simulink model "hummel_and_hubbard"  (R2021b)
settings: Solver=VariableStepAuto  StartTime=0.0  StopTime=10.0  RelTol=1e-3
values from neighbouring files (symbols this model uses):
  amb = evalin( 'base', 'amb')    [flatball_6dof_eqom.m]
  C = evalin( 'base', 'C')    [flatball_6dof_eqom.m]
  disc = evalin( 'base', 'disc')    [flatball_6dof_eqom.m]    (also in flatball_6dof_init.m = struct; flatball_init_disc_params.m = struct)
  Y0 = [0 0 -1, 0 15*C.DEG2RAD 0, 15 0 0, 0 0 (2*15*0.29/disc.d)]    [flatball_6dof_eqom.m]
libraries: simulink x4, aerolibanim x2, aerolibnav x2, matrix_library x2, mspfiltlib x1
(part 2 of 3)

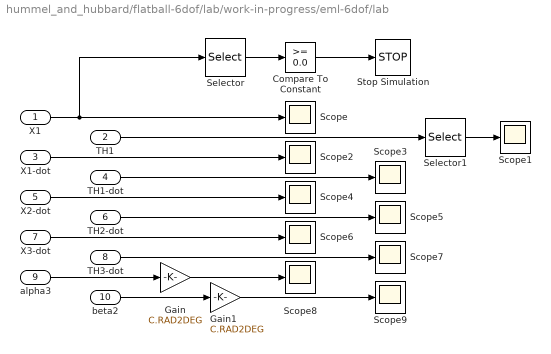
== system hummel_and_hubbard/flatball-6dof/lab/work-in-progress/eml-6dof/lab ==
  X1 : Inport
  TH1 : Inport  Port=2
  X1-dot : Inport  Port=3
  TH1-dot : Inport  Port=4
  X2-dot : Inport  Port=5
  TH2-dot : Inport  Port=6
  X3-dot : Inport  Port=7
  TH3-dot : Inport  Port=8
  alpha3 : Inport  Port=9
  beta2 : Inport  Port=10
  Compare To Constant : simulink/Logic and Bit Operations/Compare To Constant  relop=>=  const=0.0  OutDataTypeStr=boolean
  Gain : Gain  Gain=C.RAD2DEG
  Gain1 : Gain  Gain=C.RAD2DEG
  Scope{,1..9} (10 alike) : Scope
  Selector : Selector  InputPortWidth=3  IndexOptions=Index vector (dialog)  Indices=[3]  OutputSizes=1
  Selector1 : Selector  InputPortWidth=3  IndexOptions=Index vector (dialog)  Indices=[1 2]  OutputSizes=1
  Stop Simulation : Stop
  wires:
  alpha3/1 -> Gain/1
  X1-dot/1 -> Scope2/1
  X3-dot/1 -> Scope6/1
  beta2/1 -> Gain1/1
  X1/1 -> Selector/1, Scope/1
  TH1/1 -> Selector1/1
  X2-dot/1 -> Scope4/1
  TH2-dot/1 -> Scope5/1
  TH1-dot/1 -> Scope3/1
  TH3-dot/1 -> Scope7/1
  Compare To Constant/1 -> Stop Simulation/1
  Selector/1 -> Compare To Constant/1
  Gain/1 -> Scope8/1
  Gain1/1 -> Scope9/1
  Selector1/1 -> Scope1/1

== system hummel_and_hubbard/flatball-6dof/calc-F-M/lab/calc-F/aero-coeff/Subsystem ==
  alpha : Inport
  Cd0 : Constant  Value=disc.CD0
  Cda : Constant  Value=disc.CDa
  Product : Product
  Square : Math  Operator=square  SaturateOnIntegerOverflow=on
  Sum : Sum
  Sum1 : Sum
  alpha0 : Constant  Value=disc.alpha0
  Cd : Outport
  wires:
  Sum1/1 -> Cd/1
  Square/1 -> Product/2
  Product/1 -> Sum1/2
  Cda/1 -> Product/1
  Cd0/1 -> Sum1/1
  Sum/1 -> Square/1
  alpha0/1 -> Sum/2
  alpha/1 -> Sum/1

== system hummel_and_hubbard/flatball-6dof/calc-F-M/lab/calc-F/aero-coeff/Subsystem1 ==
  alpha : Inport
  CL0 : Constant  Value=disc.CL0
  CLa : Constant  Value=disc.CLa
  Product : Product
  Sum1 : Sum
  Cl : Outport
  wires:
  alpha/1 -> Product/2
  CL0/1 -> Sum1/1
  CLa/1 -> Product/1
  Product/1 -> Sum1/2
  Sum1/1 -> Cl/1

== system hummel_and_hubbard/flatball-6dof/calc-F-M/lab/calc-M/aero-coeff/Subsystem2 ==
  alpha : Inport
  CM0 : Constant  Value=disc.CM0
  CMa : Constant  Value=disc.CMa
  Product : Product
  Sum1 : Sum
  Cm : Outport
  wires:
  Sum1/1 -> Cm/1
  Product/1 -> Sum1/2
  CMa/1 -> Product/1
  CM0/1 -> Sum1/1
  alpha/1 -> Product/2

== system hummel_and_hubbard/flatball-6dof/calc-F-M/lab/helpers/Subsystem1/transformation-matrices ==
  TH : Inport
  Ta : MATLAB Function  TreatAsAtomicUnit=on
  Tr : MATLAB Function  TreatAsAtomicUnit=on
  Ta12 : Outport
  Tr12 : Outport  Port=2
  wires:
  TH/1 -> Ta/1(TH), Tr/1(TH)
  Ta/1(M) -> Ta12/1  "Ta12"
  Tr/1(M) -> Tr12/1  "Tr12"

== system hummel_and_hubbard/flatball-6dof/calc-F-M/lab/wrk/c&p/Subsystem1 ==
  X1_dot : Inport
  TH1 : Inport  Port=2
  TH1_dot : Inport  Port=3
  MatrixMultiply : Product  Multiplication=Matrix(*)
  MatrixMultiply1 : Product  Multiplication=Matrix(*)
  Transpose : Math  Operator=transpose  SaturateOnIntegerOverflow=on
  Transpose1 : Math  Operator=transpose  SaturateOnIntegerOverflow=on
  transformation-matrices : Subsystem
  w_ : MATLAB Function  TreatAsAtomicUnit=on
  TH2_dot : Outport
  w~ : Outport  Port=2
  X2_dot : Outport  Port=3
  Ta12 : Outport  Port=4
  wires:
  MatrixMultiply/1 -> X2_dot/1
  MatrixMultiply1/1 -> w_/1(THdot), TH2_dot/1
  transformation-matrices/1(Ta12) -> Transpose/1, Ta12/1
  transformation-matrices/2(Tr12) -> Transpose1/1
  X1_dot/1 -> MatrixMultiply/2
  TH1_dot/1 -> MatrixMultiply1/2
  TH1/1 -> transformation-matrices/1(TH)
  w_/1(M) -> w~/1  "w_"
  Transpose/1 -> MatrixMultiply/1  "Ta21"
  Transpose1/1 -> MatrixMultiply1/1  "Ta21"

== system hummel_and_hubbard/flatball-6dof/calc-F-M/lab/wrk/c&p/aero-coeff ==
  alpha : Inport
  Subsystem : Subsystem
  Subsystem1 : Subsystem
  Subsystem2 : Subsystem
  Cd : Outport
  Cl : Outport  Port=2
  Cm : Outport  Port=3
  wires:
  alpha/1 -> Subsystem2/1(alpha), Subsystem1/1(alpha), Subsystem/1(alpha)
  Subsystem2/1(Cm) -> Cm/1
  Subsystem1/1(Cl) -> Cl/1
  Subsystem/1(Cd) -> Cd/1

== system hummel_and_hubbard/flatball-6dof/calc-F-M/lab/wrk/c&p/q-inf ==
  x1dt : Inport
  Gain : Gain  Gain=0.5
  Product1 : Product  Inputs=3
  S : Constant  Value=disc.A
  Square : Math  Operator=square  SaturateOnIntegerOverflow=on
  rho : Constant  Value=amb.rho
  vector-norm : MATLAB Function  TreatAsAtomicUnit=on
  q-inf-S : Outport
  wires:
  Product1/1 -> Gain/1
  rho/1 -> Product1/3
  x1dt/1 -> vector-norm/1(vec)
  vector-norm/1(norm) -> Square/1
  S/1 -> Product1/2
  Square/1 -> Product1/1
  Gain/1 -> q-inf-S/1

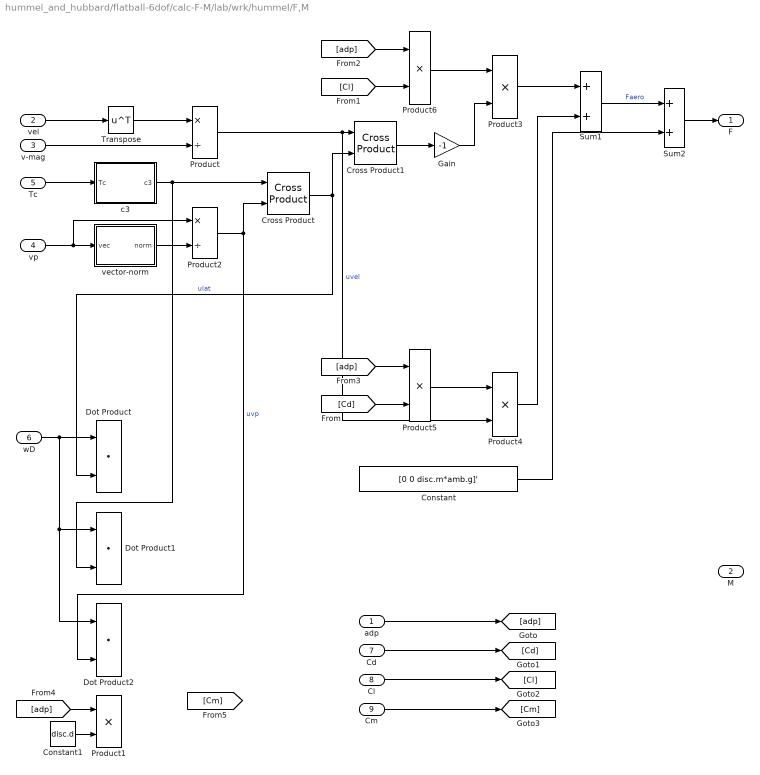
== system hummel_and_hubbard/flatball-6dof/calc-F-M/lab/wrk/hummel/F,M ==
  adp : Inport
  vel : Inport  Port=2
  v-mag : Inport  Port=3
  vp : Inport  Port=4
  Tc : Inport  Port=5
  wD : Inport  Port=6
  Cd : Inport  Port=7
  Cl : Inport  Port=8
  Cm : Inport  Port=9
  Constant : Constant  Value=[0 0 disc.m*amb.g]'
  Constant1 : Constant  Value=disc.d
  Cross Product : matrix_library/Cross Product
      settings: SourceProductBaseCode=SL
  Cross Product1 : matrix_library/Cross Product
      settings: SourceProductBaseCode=SL
  Dot Product : DotProduct  InputSameDT=on  OutDataTypeStr=Inherit: Inherit via internal rule
  Dot Product1 : DotProduct  InputSameDT=on  OutDataTypeStr=Inherit: Inherit via internal rule
  Dot Product2 : DotProduct  InputSameDT=on  OutDataTypeStr=Inherit: Inherit via internal rule
  Gain : Gain  Gain=-1
  Product : Product  Inputs=*/
  Product1 : Product  Inputs=**
  Product2 : Product  Inputs=*/
  Product{3..6} (4 alike) : Product
  Sum1 : Sum
  Sum2 : Sum
  Transpose : Math  Operator=transpose  SaturateOnIntegerOverflow=on
  c3 : MATLAB Function  TreatAsAtomicUnit=on
  vector-norm : MATLAB Function  TreatAsAtomicUnit=on
  F : Outport
  M : Outport  Port=2
  wires:
  vel/1 -> Transpose/1
  v-mag/1 -> Product/2
  vp/1 -> Product2/1, vector-norm/1(vec)
  vector-norm/1(norm) -> Product2/2
  Product2/1 -> Dot Product2/2, Cross Product/2  "uvp"
  Tc/1 -> c3/1(Tc)
  c3/1(c3) -> Dot Product1/2, Cross Product/1
  Cross Product/1 -> Cross Product1/2, Dot Product/2  "ulat"
  Product/1 -> Cross Product1/1, Product4/2  "uvel"
  Cross Product1/1 -> Gain/1
  Gain/1 -> Product3/2
  Product3/1 -> Sum1/1
  Product4/1 -> Sum1/2
  Sum1/1 -> Sum2/1  "Faero"
  Transpose/1 -> Product/1
  Sum2/1 -> F/1
  Constant/1 -> Sum2/2
  adp/1 -> [adp]
  Constant1/1 -> Product1/2
  wD/1 -> Dot Product2/1, Dot Product1/1, Dot Product/1
  Product5/1 -> Product4/1
  [Cl] -> Product6/2
  [Cd] -> Product5/2
  Product6/1 -> Product3/1
  [adp] -> Product6/1
  [adp] -> Product5/1
  Cd/1 -> [Cd]
  Cl/1 -> [Cl]
  Cm/1 -> [Cm]
  [adp] -> Product1/1

== system hummel_and_hubbard/flatball-6dof/calc-F-M/lab/wrk/hummel/Radv ==
  v-mag : Inport
  TH-dt : Inport  Port=2
  Gain : Gain  Gain=0.5
  Product1 : Product  Inputs=**/
  Selector : Selector  InputPortWidth=3  IndexOptions=Index vector (dialog)  Indices=[3]  OutputSizes=1
  "[0.5 .. inf]" : Saturate  UpperLimit=inf  LowerLimit=0.50
  d : Constant  Value=disc.d
  Radv : Outport
  wires:
  Product1/1 -> Radv/1
  d/1 -> Gain/1
  TH-dt/1 -> Selector/1
  Selector/1 -> Product1/1
  Gain/1 -> Product1/2
  v-mag/1 -> "[0.5 .. inf]"/1
  "[0.5 .. inf]"/1 -> Product1/3

== system hummel_and_hubbard/flatball-6dof/calc-F-M/lab/wrk/hummel/Subsystem ==
  phi : Inport
  theta : Inport  Port=2
  Tc : MATLAB Function  TreatAsAtomicUnit=on
  T : Outport
  wires:
  theta/1 -> Tc/2(theta)
  phi/1 -> Tc/1(phi)
  Tc/1(Tc) -> T/1

== system hummel_and_hubbard/flatball-6dof/calc-F-M/lab/wrk/hummel/adp ==
  v-mag : Inport
  A : Constant  Value=disc.A
  Gain : Gain  Gain=0.5
  Product : Product
  Product1 : Product  Inputs=3
  rho : Constant  Value=amb.rho
  adp : Outport
  wires:
  Product1/1 -> adp/1
  rho/1 -> Product/1
  A/1 -> Product/2
  Product/1 -> Gain/1
  v-mag/1 -> Product1/2, Product1/1
  Gain/1 -> Product1/3

== system hummel_and_hubbard/flatball-6dof/calc-F-M/lab/wrk/hummel/aero-coeff ==
  alpha : Inport
  Subsystem : Subsystem
  Subsystem1 : Subsystem
  Subsystem2 : Subsystem
  Cd : Outport
  Cl : Outport  Port=2
  Cm : Outport  Port=3
  wires:
  alpha/1 -> Subsystem2/1(alpha), Subsystem1/1(alpha), Subsystem/1(alpha)
  Subsystem2/1(Cm) -> Cm/1
  Subsystem1/1(Cl) -> Cl/1
  Subsystem/1(Cd) -> Cd/1

== system hummel_and_hubbard/flatball-6dof/calc-F-M/lab/wrk/c&p/Subsystem1/transformation-matrices ==
  TH : Inport
  Ta : MATLAB Function  TreatAsAtomicUnit=on
  Tr : MATLAB Function  TreatAsAtomicUnit=on
  Ta12 : Outport
  Tr12 : Outport  Port=2
  wires:
  TH/1 -> Ta/1(TH), Tr/1(TH)
  Ta/1(Ta12) -> Ta12/1
  Tr/1(Tr12) -> Tr12/1

== system hummel_and_hubbard/flatball-6dof/calc-F-M/lab/wrk/c&p/aero-coeff/Subsystem ==
  alpha : Inport
  Cd0 : Constant  Value=disc.CD0
  Cda : Constant  Value=disc.CDa
  Product : Product
  Square : Math  Operator=square  SaturateOnIntegerOverflow=on
  Sum : Sum
  Sum1 : Sum
  alpha0 : Constant  Value=disc.alpha0
  Cd : Outport
  wires:
  Sum1/1 -> Cd/1
  Square/1 -> Product/2
  Product/1 -> Sum1/2
  Cda/1 -> Product/1
  Cd0/1 -> Sum1/1
  Sum/1 -> Square/1
  alpha0/1 -> Sum/2
  alpha/1 -> Sum/1

== system hummel_and_hubbard/flatball-6dof/calc-F-M/lab/wrk/c&p/aero-coeff/Subsystem1 ==
  alpha : Inport
  CL0 : Constant  Value=disc.CL0
  CLa : Constant  Value=disc.CLa
  Product : Product
  Sum1 : Sum
  Cl : Outport
  wires:
  alpha/1 -> Product/2
  CL0/1 -> Sum1/1
  CLa/1 -> Product/1
  Product/1 -> Sum1/2
  Sum1/1 -> Cl/1

== system hummel_and_hubbard/flatball-6dof/calc-F-M/lab/wrk/c&p/aero-coeff/Subsystem2 ==
  alpha : Inport
  CM0 : Constant  Value=disc.CM0
  CMa : Constant  Value=disc.CMa
  Product : Product
  Sum1 : Sum
  Cm : Outport
  wires:
  Sum1/1 -> Cm/1
  Product/1 -> Sum1/2
  CMa/1 -> Product/1
  CM0/1 -> Sum1/1
  alpha/1 -> Product/2

== system hummel_and_hubbard/flatball-6dof/calc-F-M/lab/wrk/hummel/aero-coeff/Subsystem ==
  alpha : Inport
  Cd0 : Constant  Value=disc.CD0
  Cda : Constant  Value=disc.CDa
  Product : Product
  Square : Math  Operator=square  SaturateOnIntegerOverflow=on
  Sum : Sum
  Sum1 : Sum
  alpha0 : Constant  Value=disc.alpha0
  Cd : Outport
  wires:
  Sum1/1 -> Cd/1
  Square/1 -> Product/2
  Product/1 -> Sum1/2
  Cda/1 -> Product/1
  Cd0/1 -> Sum1/1
  Sum/1 -> Square/1
  alpha0/1 -> Sum/2
  alpha/1 -> Sum/1

== system hummel_and_hubbard/flatball-6dof/calc-F-M/lab/wrk/hummel/aero-coeff/Subsystem1 ==
  alpha : Inport
  CL0 : Constant  Value=disc.CL0
  CLa : Constant  Value=disc.CLa
  Product : Product
  Sum1 : Sum
  Cl : Outport
  wires:
  alpha/1 -> Product/2
  CL0/1 -> Sum1/1
  CLa/1 -> Product/1
  Product/1 -> Sum1/2
  Sum1/1 -> Cl/1

== system hummel_and_hubbard/flatball-6dof/calc-F-M/lab/wrk/hummel/aero-coeff/Subsystem2 ==
  alpha : Inport
  CM0 : Constant  Value=disc.CM0
  CMa : Constant  Value=disc.CMa
  Product : Product
  Sum1 : Sum
  Cm : Outport
  wires:
  Sum1/1 -> Cm/1
  Product/1 -> Sum1/2
  CMa/1 -> Product/1
  CM0/1 -> Sum1/1
  alpha/1 -> Product/2

== matlab function hummel_and_hubbard/flatball-6dof/calc-F-M/lab/helpers/Subsystem2/angle-of-attack ==
  data: Xdot input; alpha output
function alpha  = f( Xdot)
% calculate angle of attack

alpha = atan( Xdot(3) / Xdot(1));

== matlab function hummel_and_hubbard/flatball-6dof/calc-Xdot/calc-Xdot ==
  data: X input; F input; Xdot output
function Xdot   = f_lin( X, F)
% flatball equations of motion - NED (north-east-down) configuration
%

%% internal states
% x = X(1); y = X(2); z = X(3);
u = X(7); v = X(8); w = X(9);

Xdot = zeros(1,6);

%% define non-aerodynamic parameters
disc = struct;
disc.m = 0.175; % Kg

%%
    xdotdot = F(1) / disc.m;
    ydotdot = F(2) / disc.m;
    zdotdot = F(3) / disc.m;

%%
Xdot(1) = u;
Xdot(2) = v;
Xdot(3) = w;

Xdot(4) = xdotdot;
Xdot(5) = ydotdot;
Xdot(6) = zdotdot;

== matlab function hummel_and_hubbard/flatball-6dof/calc-F-M/lab/wrk/hummel/vector-norm ==
  data: vec input; norm output
function norm = fcn( vec)

norm = sqrt( vec(1)*vec(1) + vec(2)*vec(2) + vec(3)*vec(3));

== matlab function hummel_and_hubbard/flatball-6dof/calc-F-M/lab/wrk/hummel/Subsystem/Tc ==
  data: phi input; theta input; Tc output
function Tc = fcn( phi, theta)

sin_theta = sin( theta);
cos_theta = cos( theta);
sin_phi = sin( phi);
cos_phi = cos(phi);

Tc = [
    cos_theta sin_theta*sin_phi -sin_theta*cos_phi;
    0 cos_phi sin_phi;
    sin_theta -cos_theta*sin_phi cos_theta*cos_phi;
    ];

== matlab function hummel_and_hubbard/flatball-6dof/calc-F-M/lab/wrk/hummel/vp ==
  data: vel input; vp output; Tc input; vc3 input
function vp = fcn( vel, Tc, vc3)

c3 = Tc(:,3);

vp = [ vel - vc3*c3];

== matlab function hummel_and_hubbard/flatball-6dof/calc-F-M/lab/wrk/hummel/alpha ==
  data: v_N input; vc3 input; alpha output
function alpha = fcn( v_N, vc3)

alpha = atan( vc3 / norm( v_N)); % angle of attack

== matlab function hummel_and_hubbard/flatball-6dof/calc-F-M/lab/wrk/hummel/vc3 ==
  data: vel input; vc3 output; Tc input
function vc3 = fcn( vel, Tc)

c3 = Tc(:,3);
vc3 = dot( vel, c3);

== matlab function hummel_and_hubbard/flatball-6dof/calc-F-M/lab/wrk/c&p/Ta ==
  data: beta input; T output
function T  = Ta23( beta)
% transformation matrix
%

cos_beta = cos( beta);
sin_beta = sin( beta);

T = [ ...
    cos_beta -sin_beta 0;
    -sin_beta cos_beta 0;
    0 0 1;
    ];

== matlab function hummel_and_hubbard/flatball-6dof/calc-F-M/lab/wrk/hummel/F,M/vector-norm ==
  data: vec input; norm output
function norm = fcn( vec)

norm = sqrt( vec(1)*vec(1) + vec(2)*vec(2) + vec(3)*vec(3));

== matlab function hummel_and_hubbard/flatball-6dof/calc-F-M/lab/wrk/hummel/F,M/c3 ==
  data: Tc input; c3 output
function c3 = fcn( Tc)

c3 = Tc(:,3);

== matlab function hummel_and_hubbard/flatball-6dof/calc-F-M/lab/wrk/hummel/wD ==
  data: TH input; TH_dt input; wD output; Tc input
function wD = fcn( TH, TH_dt, Tc)

cos_theta = cos( TH(2));
sin_theta = sin( TH(2));

phidot = TH_dt(1);
thetadot = TH_dt(2);
gammadot = TH_dt(3);

wD_N_inC = [phidot*cos_theta thetadot phidot*sin_theta+gammadot];
wD = Tc' * wD_N_inC';

== matlab function hummel_and_hubbard/flatball-6dof/calc-F-M/lab/wrk/c&p/q-inf/vector-norm ==
  data: vec input; norm output
function norm = fcn( vec)

norm = sqrt( vec(1)*vec(1) + vec(2)*vec(2) + vec(3)*vec(3));

== matlab function hummel_and_hubbard/flatball-6dof/calc-F-M/lab/wrk/c&p/Subsystem1/transformation-matrices/Ta ==
  data: TH input; Ta12 output
function Ta12  = Ta( TH)
% transformation matrix
%
phi = TH(1); theta = TH(2); psi = TH(3);

cos_phi = cos( phi);
cos_theta = cos( theta);
cos_psi = cos( psi);

sin_phi = sin( phi);
sin_theta = sin( theta);
sin_psi = sin( psi);

Ta12 = [ ...
    cos_theta*cos_psi sin_phi*sin_theta*cos_phi-cos_phi*sin_psi cos_phi*sin_theta*cos_psi+sin_phi*sin_psi;
    cos_theta*sin_psi sin_phi*sin_theta*sin_psi+cos_phi*cos_psi cos_phi*sin_theta*sin_psi-sin_phi*cos_psi;
    -sin_theta sin_phi*cos_theta cos_phi*cos_theta
    ];

% cos_neg_phi = cos( -phi);
% cos_neg_theta = cos( -theta);
% cos_neg_psi = cos( -psi);
% 
% sin_neg_phi = sin( -phi);
% sin_neg_theta = sin( -theta);
% sin_neg_psi = sin( -psi);
% 
% Ta12 = [ ...
%     cos_neg_theta*cos_neg_psi sin_neg_phi*sin_neg_theta*cos_neg_phi-cos_neg_phi*sin_neg_psi cos_neg_phi*sin_neg_theta*cos_neg_psi+sin_neg_phi*sin_neg_psi;
%     cos_neg_theta*sin_neg_psi sin_neg_phi*sin_neg_theta*sin_neg_psi+cos_neg_phi*cos_neg_psi cos_neg_phi*sin_neg_theta*sin_neg_psi-sin_neg_phi*cos_neg_psi;
%     -sin_neg_theta sin_neg_phi*cos_neg_theta cos_neg_phi*cos_neg_theta
%     ];

== matlab function hummel_and_hubbard/flatball-6dof/calc-F-M/lab/wrk/c&p/Subsystem1/transformation-matrices/Tr ==
  data: TH input; Tr12 output
function Tr12  = Tr( TH)
% transformation matrix
%
phi = TH(1); theta = TH(2); psi = TH(3);

cos_phi = cos( phi);
cos_theta = cos( theta);
cos_psi = cos( psi);

sin_phi = sin( phi);
sin_theta = sin( theta);
sin_psi = sin( psi);

Tr12 = [
    1 0 -sin_theta;
    0 cos_phi cos_theta*sin_psi;
    0 -sin_phi cos_theta*cos_psi;
    ];

== matlab function hummel_and_hubbard/flatball-6dof/calc-F-M/lab/wrk/c&p/Subsystem1/w_ ==
  data: THdot input; M output
function M  = w_( THdot)
% transformation matrix
%
p = THdot(1); q = THdot(2); r = THdot(3);

M = [ ...
    0 -r q;
    r 0 -p;
    -q p 0
    ];

== matlab function hummel_and_hubbard/flatball-6dof/calc-F-M/lab/wrk/c&p/Ta1 ==
  data: alpha input; T output
function T  = Ta34( alpha)
% transformation matrix
%

cos_alpha = cos( alpha);
sin_alpha = sin( alpha);

T= [ ...
    cos_alpha 0 -sin_alpha;
    0 1 0;
    sin_alpha 0 cos_alpha;
    ];

== matlab function hummel_and_hubbard/flatball-6dof/calc-F-M/lab/wrk/c&p/angle-of-attack ==
  data: Xdot input; alpha output
function alpha  = f( Xdot)
% calculate angle of attack

alpha = atan2( Xdot(3) / Xdot(1));

== matlab function hummel_and_hubbard/flatball-6dof/calc-F-M/lab/wrk/c&p/zero-side-slip-angle ==
  data: Xdot input; beta output
function beta  = f( Xdot)
% calculate side-slip angle

y = Xdot(2);
x = Xdot(1);

beta = atan2( y / x);

== matlab function hummel_and_hubbard/flatball-6dof/calc-F-M/lab/wrk/flatball_6dof_v1p1 ==
  data: X input; Xdot output; lift output; drag output; alpha output; AdvR output; E_trans output; E_rot output
function [Xdot, lift, drag, alpha, AdvR, E_trans, E_rot]  = flatball_6dof_eom( X)
% flatball equations of motion - NED (north-east-down) configuration
%

%% internal states
x = X(1); y = X(2); z = X(3);
xdot = X(4); ydot = X(5); zdot = X(6);

phi = X(7); theta = X(8); gamma = X(9);
phidot = X(10); thetadot = X(11); gammadot = X(12);

Xdot = zeros(1,12);

%% define ambient parameters
amb.g = 9.81; % m/s^2
amb.rho = 1.23; % Kg/m^3

%% define non-aerodynamic parameters
disc = struct;
disc.m = 0.175; % Kg
disc.A = 0.057; % m^2
disc.d = 2*sqrt(0.057/pi); % 2*sqrt(disc.A/pi); % diameter
disc.Ia = 0.002352; % moment of inertia about the spinning axis
disc.Id = 0.001219; % moment of inertia about the planar axis'

%% crowther and potts - per hummel and hubbard
% disc.CL0 = 0.13;
% disc.CLa = 3.09;
% disc.CD0 = 0.085;
% disc.CDa = 3.30;
% disc.CM0 = -0.01;
% disc.CMa = 0.057;
% 
% disc.CMq = 0.0008; % NOTE: not used
% disc.CLr = 0.0004;
% disc.CLp = -0.013;
% disc.CNr = -2.8e-5;
% 
% disc.alpha0 = -0.052; % rad

%% hummel and hubbard 2014
disc.CL0 = 0.188;
disc.CLa = 2.37;

disc.CD0 = 0.15;
disc.CDa = 1.24;

disc.CM0 = -0.06;
disc.CMa = 0.38;

disc.CMq = 0.0008; % NOTE: not used
disc.CLr = 0.0004;

disc.CNr = -2.8e-5;

disc.CLp = -0.013;

% disc.CRr = 1.4e-2; % NOTE: missing from 2014, borrowed from 2003 thesis
% disc.CRr = 3e-3; % NOTE: missing from 2014, borrowed from P&C
disc.CRr = 0.00171; % appendix of hummel thesis
disc.CRp =-5.5e-3; % NOTE: missing from 2014, borrowed from P&C

% not sure where these are from...
% disc.CMq= -1.44E-02;
% disc.CRp =-1.25E-02;
% disc.CNr = -3.41E-05; % long flight f2302

disc.alpha0 = -0.052; % rad

%% helper variables
sin_theta = sin( theta);
cos_theta = cos( theta);
sin_phi = sin( phi);
cos_phi = cos(phi);

% c = T_c_N * N --> transformation matrix T_c_N in N reference frame
T_c_N = [cos_theta sin_theta*sin_phi -sin_theta*cos_phi;
    0 cos_phi sin_phi;
    sin_theta -cos_theta*sin_phi cos_theta*cos_phi];
% c1 = T_c_N(1,:);
% c2 = T_c_N(2,:);
c3 = T_c_N(3,:);

%% aerodynamic forces and moments in N reference frame
vel = [xdot ydot zdot];
vmag = norm( vel);
vc3 = dot( vel, c3);
v_N = [ vel - vc3*c3];
Adp = 0.5 * disc.A * amb.rho * vmag*vmag;
uvel = vel / vmag;
uv_N = v_N / norm( v_N);
u_lat = cross( c3, uv_N);

wD_N_inC = [phidot*cos_theta thetadot phidot*sin_theta+gammadot];
wD_N_inN = T_c_N' * wD_N_inC';

w_v_N = dot( wD_N_inN, uv_N);
w_lat = dot( wD_N_inN, u_lat);
w_spin = dot( wD_N_inN, c3);

alpha = atan( vc3 / norm( v_N)); % angle of attack
AdvR = disc.d * w_spin / 2 / vmag; % advance ratio
E_trans = 0.5 * disc.m * vmag*vmag; % translational energy
E_rot = 0.5 * disc.Ia * gammadot*gammadot; % rotational energy

%% hacks
k_spin_down_decay = 0.25;
% k_CL_gain = 1.0; %2.5;
% k_CD_gain = 1.0; %1.5;
% k_M_gain = 1.0;

%% coefficients - f(alpha)
dalpha = alpha - disc.alpha0;
CL = disc.CL0 + disc.CLa * alpha;
CD = disc.CD0 + disc.CDa * dalpha*dalpha;
CM = disc.CM0 + disc.CMa * alpha;
Mv_N = Adp * disc.d * (sqrt(disc.d/amb.g)*disc.CRr*w_spin + disc.CRp*w_v_N) * uv_N;

%% coefficients - lookup based
% 
% CL = interp1( disc.CL_data(:,1), disc.CL_data(:,2).*k_CL_gain, alpha, 'spline');
% CD = interp1( disc.CD_data(:,1), disc.CD_data(:,2).*k_CD_gain, alpha, 'spline');
% CM = interp1( disc.CM_data(:,1), disc.CM_data(:,2).*k_M_gain, alpha, 'spline');
% % CRr = interp2( disc.CRr_rad, disc.CRr_AdvR, disc.CRr_data, alpha, AdvR,'spline');
% Mv_N = Adp * disc.d * ( disc.CRr* + disc.CRp*w_v_N) * uv_N;

%%
lift = CL * Adp;
drag = CD * Adp;
ulift = -cross( uvel, u_lat);
udrag = -uvel;
Faero = lift*ulift + drag*udrag;
Fg_N = [0 0 disc.m*amb.g]';

F = Faero' + Fg_N;

Mlat = Adp * disc.d * (CM + disc.CMq * w_lat) * u_lat;
Mspin = [0 0 disc.CNr*w_spin];
M = T_c_N * Mv_N' + T_c_N*Mlat' + Mspin';

%%
xdotdot = F(1) / disc.m;
ydotdot = F(2) / disc.m;
zdotdot = F(3) / disc.m;

phidotdot = (M(1) + disc.Id*thetadot*phidot*sin_theta - disc.Ia*thetadot*(phidot*sin_theta+gammadot) + disc.Id*thetadot*phidot*sin_theta)/disc.Id/cos_theta; 
thetadotdot = (M(2) + disc.Ia*phidot*cos_theta*(phidot*sin_theta +gammadot) - disc.Id*phidot*phidot*cos_theta*sin_theta)/disc.Id;
gammadotdot = (M(3) - disc.Ia*(k_spin_down_decay*gammadot*sin_theta + thetadot*phidot*cos_theta))/disc.Ia;

% bug in hummels report?
% gammadotdot = (M(3) - disc.Ia*(phidotdot*sin_theta + thetadot*phidot*cos_theta))/disc.Ia;
% bug in hummels report?
% w/phidotdot term, there is no decay in gammadot
% w/out gammadot term - there is no decay in gammadot
% NOTE: w/it, the decay is too agressive
% FIXME: investigate why this term is necessary for more appropriate
% spindown (based on my data)

%%
Xdot(1) = xdot;
Xdot(2) = ydot;
Xdot(3) = zdot;

Xdot(4) = xdotdot;
Xdot(5) = ydotdot;
Xdot(6) = zdotdot;

Xdot(7) = phidot;
Xdot(8) = thetadot;
Xdot(9) = gammadot;

Xdot(10) = phidotdot;
Xdot(11) = thetadotdot;
Xdot(12) = gammadotdot;

== matlab function hummel_and_hubbard/flatball-6dof/calc-F-M/lab/rotations/X-to-T_c_N ==
  data: X input; T_c_N output
function T_c_N  = f( X)
%% internal states
phi = X(7); theta = X(8);

%% helper variables
sin_theta = sin( theta);
cos_theta = cos( theta);
sin_phi = sin( phi);
cos_phi = cos(phi);

T_c_N = [
    cos_theta sin_theta*sin_phi -sin_theta*cos_phi;
    0 cos_phi sin_phi;
    sin_theta -cos_theta*sin_phi cos_theta*cos_phi
    ];

== matlab function hummel_and_hubbard/flatball-6dof/calc-F-M/lab/alpha- ==
  data: X input; alpha output; T_c_N input
function alpha  = f( X, T_c_N)
%% internal states
xdot = X(4); ydot = X(5); zdot = X(6);

%% helper variables
T_c_Npsi = T_c_N(3,:);

vel = [xdot ydot zdot];
vc3 = dot( vel, T_c_Npsi);
v_N = [ vel - vc3*T_c_Npsi];

alpha = atan( vc3 / norm( v_N)); % angle of attack

== matlab function hummel_and_hubbard/flatball-6dof/calc-F-M/lab/rotations/X-to-wD_N_inC ==
  data: X input; wD_N_inC output
function wD_N_inC  = f( X)
%% internal states
theta = X(8);
phidot = X(10); thetadot = X(11); gammadot = X(12);

%% helper variables
sin_theta = sin( theta);
cos_theta = cos( theta);

wD_N_inC = [phidot*cos_theta thetadot phidot*sin_theta+gammadot];

== matlab function hummel_and_hubbard/flatball-6dof/calc-F-M/lab/calc-F/q-inf/vector-norm ==
  data: vec input; norm output
function norm = fcn( vec)

norm = sqrt( vec(1)*vec(1) + vec(2)*vec(2) + vec(3)*vec(3));

== matlab function hummel_and_hubbard/flatball-6dof/calc-F-M/lab/calc-F/q-inf/X-to-vel ==
  data: X input; vel output
function vel = fcn( X)
xdot = X(4); ydot = X(5); zdot = X(6);
vel = [xdot ydot zdot];

== matlab function hummel_and_hubbard/flatball-6dof/calc-F-M/lab/calc-F/X-to-vel ==
  data: X input; vel output
function vel = fcn( X)
xdot = X(4); ydot = X(5); zdot = X(6);
vel = [xdot ydot zdot];

== matlab function hummel_and_hubbard/flatball-6dof/calc-F-M/lab/calc-M/X-to-vel ==
  data: X input; vel output
function vel = fcn( X)
xdot = X(4); ydot = X(5); zdot = X(6);
vel = [xdot ydot zdot];

== matlab function hummel_and_hubbard/flatball-6dof/calc-F-M/lab/calc-F/calc-F ==
  data: vel input; F output; T_c_N input; Fg_N input; CLift input; CDrag input; q_inf_times_S input
function F = fcn( vel, T_c_N, Fg_N, CLift, CDrag, q_inf_times_S)
%%
T_c_Npsi = T_c_N(3,:);

vc3 = dot( vel, T_c_Npsi);
v_N = [ vel - vc3*T_c_Npsi];
vmag = norm( vel);
uvel = vel / vmag;
uv_N = v_N / norm( v_N);
u_lat = cross( T_c_Npsi, uv_N);

lift = CLift * q_inf_times_S;
ulift = -cross( uvel, u_lat);

drag = CDrag * q_inf_times_S;
udrag = -uvel;

Faero = lift*ulift + drag*udrag;

F = Faero' + Fg_N;

== matlab function hummel_and_hubbard/flatball-6dof/calc-F-M/lab/wrk/flatball_6dof_v1p0 ==
  data: X input; Xdot output; lift output; drag output; alpha output; AdvR output; E_trans output; E_rot output
function [Xdot, lift, drag, alpha, AdvR, E_trans, E_rot]  = flatball_6dof_eom( X)
% flatball equations of motion - NED (north-east-down) configuration
%

%% internal states
x = X(1); y = X(2); z = X(3);
xdot = X(4); ydot = X(5); zdot = X(6);

phi = X(7); theta = X(8); gamma = X(9);
phidot = X(10); thetadot = X(11); gammadot = X(12);

Xdot = zeros(1,12);

%% define ambient parameters
amb.g = 9.81; % m/s^2
amb.rho = 1.23; % Kg/m^3

%% define non-aerodynamic parameters
disc = struct;
disc.m = 0.175; % Kg
disc.A = 0.057; % m^2
disc.d = 2*sqrt(0.057/pi); % 2*sqrt(disc.A/pi); % diameter
disc.Ia = 0.002352; % moment of inertia about the spinning axis
disc.Id = 0.001219; % moment of inertia about the planar axis'

disc.alpha0 = -0.052; %-4 * pi/180.0;

%% THE THREE ESTIMATED COEFFICIENTS
disc.CMq= -1.44E-02;
disc.CRp =-1.25E-02;
disc.CNr = -3.41E-05; % long flight f2302

%% THE seven COEFFICIENTS estimated from three flights
disc.CL0= 0.13; %c&p 07
disc.CLa= 3.09; %c&p 07
disc.CD0= 0.085; %c&p 07
disc.CDa= 3.30; %c&p 07
disc.CM0= -0.01; %c&p 07
disc.CMa= 0.057; %c&p 07 
disc.CRr= 0.00171; % for nondimensionalization = sqrt(d/g), magnitude of CRr changes

%% CL =[ rad CL deg]
disc.CL_data=[ -0.1745 -0.2250 -10; ...
-0.05236 0 -3; ...
0 0.150 0; ...
0.08727 0.4500 5; ...
0.17453 0.7250 10; ...
0.26180 0.9750 15; ...
0.34907 1.2000 20; ...
0.43633 1.4500 25; ...
0.52360 1.6750 30];

%% CD =[ rad CD deg]
disc.CD_data=[ -0.1745 0.1500 -10; ...
-0.05236 0.0800 -3; ...
0 0.1000 0; ...
0.08727 0.1500 5; ...
0.1745 0.2600 10; ...
0.26180 0.3900 15; ...
0.3491 0.5700 20; ...
0.4363 0.7500 25; ...
0.5236 0.9200 30];

%% CM =[ rad CM deg]
disc.CM_data=[-0.174532925 -0.0380 -10; ...
-0.087266463 -0.0220 -5; ...
-0.052359878 -0.0140 -3; ...
0 -0.0060 0; ...
0.052359878 -0.0060 3; ...
0.104719755 -0.0020 6; ...
0.157079633 0.0000 9; ...
0.20943951 0.0100 12; ...
0.261799388 0.0220 15; ...
0.34906585 0.0440 20; ...
0.401425728 0.0600 23; ...
0.453785606 0.0840 26; ...
0.523598776 0.1100 30];

%% helper variables
sin_theta = sin( theta);
cos_theta = cos( theta);
sin_phi = sin( phi);
cos_phi = cos(phi);

% c = T_c_N * N --> transformation matrix T_c_N in N reference frame
T_c_N = [cos_theta sin_theta*sin_phi -sin_theta*cos_phi;
    0 cos_phi sin_phi;
    sin_theta -cos_theta*sin_phi cos_theta*cos_phi];
% c1 = T_c_N(1,:);
% c2 = T_c_N(2,:);
c3 = T_c_N(3,:);

%% aerodynamic forces and moments in N reference frame
vel = [xdot ydot zdot];
vmag = norm( vel);
vc3 = dot( vel, c3);
v_N = [ vel - vc3*c3];
Adp = 0.5 * disc.A * amb.rho * vmag*vmag;
uvel = vel / vmag;
uv_N = v_N / norm( v_N);
u_lat = cross( c3, uv_N);

wD_N_inC = [phidot*cos_theta thetadot phidot*sin_theta+gammadot];
wD_N_inN = T_c_N' * wD_N_inC';

w_v_N = dot( wD_N_inN, uv_N);
w_lat = dot( wD_N_inN, u_lat);
w_spin = dot( wD_N_inN, c3);

alpha = atan( vc3 / norm( v_N)); % angle of attack
AdvR = disc.d * w_spin / 2 / vmag; % advance ratio
E_trans = 0.5 * disc.m * vmag*vmag; % translational energy
E_rot = 0.5 * disc.Ia * gammadot*gammadot; % rotational energy

%% hacks
k_spin_down_decay = 0.25;
% k_CL_gain = 1.0; %2.5;
% k_CD_gain = 1.0; %1.5;
% k_M_gain = 1.0;

%% coefficients - f(alpha)
dalpha = alpha - disc.alpha0;
CL = disc.CL0 + disc.CLa * alpha;
CD = disc.CD0 + disc.CDa * dalpha*dalpha;
CM = disc.CM0 + disc.CMa * alpha;
Mv_N = Adp * disc.d * (sqrt(disc.d/amb.g)*disc.CRr*w_spin + disc.CRp*w_v_N) * uv_N;

%% coefficients - lookup based
% 
% CL = interp1( disc.CL_data(:,1), disc.CL_data(:,2).*k_CL_gain, alpha, 'spline');
% CD = interp1( disc.CD_data(:,1), disc.CD_data(:,2).*k_CD_gain, alpha, 'spline');
% CM = interp1( disc.CM_data(:,1), disc.CM_data(:,2).*k_M_gain, alpha, 'spline');
% % CRr = interp2( disc.CRr_rad, disc.CRr_AdvR, disc.CRr_data, alpha, AdvR,'spline');
% Mv_N = Adp * disc.d * ( disc.CRr* + disc.CRp*w_v_N) * uv_N;

%%
lift = CL * Adp;
drag = CD * Adp;
ulift = -cross( uvel, u_lat);
udrag = -uvel;
Faero = lift*ulift + drag*udrag;
Fg_N = [0 0 disc.m*amb.g]';

F = Faero' + Fg_N;

Mlat = Adp * disc.d * (CM + disc.CMq * w_lat) * u_lat;
Mspin = [0 0 disc.CNr*w_spin];
M = T_c_N * Mv_N' + T_c_N*Mlat' + Mspin';

%%
xdotdot = F(1) / disc.m;
ydotdot = F(2) / disc.m;
zdotdot = F(3) / disc.m;

phidotdot = (M(1) + disc.Id*thetadot*phidot*sin_theta - disc.Ia*thetadot*(phidot*sin_theta+gammadot) + disc.Id*thetadot*phidot*sin_theta)/disc.Id/cos_theta; 
thetadotdot = (M(2) + disc.Ia*phidot*cos_theta*(phidot*sin_theta +gammadot) - disc.Id*phidot*phidot*cos_theta*sin_theta)/disc.Id;
gammadotdot = (M(3) - disc.Ia*(k_spin_down_decay*gammadot*sin_theta + thetadot*phidot*cos_theta))/disc.Ia;

% bug in hummels report?
% gammadotdot = (M(3) - disc.Ia*(phidotdot*sin_theta + thetadot*phidot*cos_theta))/disc.Ia;
% bug in hummels report?
% w/phidotdot term, there is no decay in gammadot
% w/out gammadot term - there is no decay in gammadot
% NOTE: w/it, the decay is too agressive
% FIXME: investigate why this term is necessary for more appropriate
% spindown (based on my data)

%%
Xdot(1) = xdot;
Xdot(2) = ydot;
Xdot(3) = zdot;

Xdot(4) = xdotdot;
Xdot(5) = ydotdot;
Xdot(6) = zdotdot;

Xdot(7) = phidot;
Xdot(8) = thetadot;
Xdot(9) = gammadot;

Xdot(10) = phidotdot;
Xdot(11) = thetadotdot;
Xdot(12) = gammadotdot;

== matlab function hummel_and_hubbard/flatball-6dof/calc-F-M/lab/calc-M/calc-M ==
  data: vel input; M output; T_c_N input; wD_N_inN input; CMpitch input; q_inf_times_Sd input
function M = fcn( vel, T_c_N, wD_N_inN, CMpitch, q_inf_times_Sd)
%% define ambient parameters
amb.g = 9.81; % m/s^2
amb.rho = 1.23; % Kg/m^3

%% define non-aerodynamic parameters
disc = struct;
disc.m = 0.175; % Kg
disc.A = 0.057; % m^2
disc.d = 2*sqrt(0.057/pi); % 2*sqrt(disc.A/pi); % diameter
disc.Ia = 0.002352; % moment of inertia about the spinning axis
disc.Id = 0.001219; % moment of inertia about the planar axis'

%% crowther and potts - per hummel and hubbard
disc.CMq= -1.44e-2;
disc.CNr = -7.1e-6; % short flights
% disc.CNr = -3.41e-5; % long flight f2302
disc.CRr = 3e-3; % NOTE: missing from 2014, borrowed from P&C
disc.CRp =-5.5e-3; % NOTE: missing from 2014, borrowed from P&C
% disc.CLr = 0.0004;
% disc.CLp = -0.013;
% 

%% helper variables
T_c_Npsi = T_c_N(3,:);

%% aerodynamic forces and moments in N reference frame
vc3 = dot( vel, T_c_Npsi);
v_N = [ vel - vc3*T_c_Npsi];

uv_N = v_N / norm( v_N);
u_lat = cross( T_c_Npsi, uv_N);

w_v_N = dot( wD_N_inN, uv_N);
q = dot( wD_N_inN, u_lat);
r = dot( wD_N_inN, T_c_Npsi);
%%
Mv_N = q_inf_times_Sd * (sqrt(disc.d/amb.g)*disc.CRr*r + disc.CRp*w_v_N) * uv_N;
Mpitch = q_inf_times_Sd * (CMpitch + disc.CMq * q) * u_lat;
Mspin = [0 0 disc.CNr*r];
M = T_c_N*Mv_N' + T_c_N*Mpitch' + Mspin';

== matlab function hummel_and_hubbard/flatball-6dof/calc-F-M/lab/calc-M/q-inf/X-to-vel ==
  data: X input; vel output
function vel = fcn( X)
xdot = X(4); ydot = X(5); zdot = X(6);
vel = [xdot ydot zdot];

== matlab function hummel_and_hubbard/flatball-6dof/calc-F-M/lab/calc-M/q-inf/vector-norm ==
  data: vec input; norm output
function norm = fcn( vec)

norm = sqrt( vec(1)*vec(1) + vec(2)*vec(2) + vec(3)*vec(3));

== matlab function hummel_and_hubbard/flatball-6dof/calc-F-M/lab/internals ==
  data: X input; AdvR output; E_trans output; E_rot output; T_c_N input; wD_N_inN input
function [ AdvR, E_trans, E_rot]  = internals( X, T_c_N, wD_N_inN)
%% internal states
x = X(1); y = X(2); z = X(3);
xdot = X(4); ydot = X(5); zdot = X(6);

phi = X(7); theta = X(8); gamma = X(9);
phidot = X(10); thetadot = X(11); gammadot = X(12);

%% define non-aerodynamic parameters
disc = struct;
disc.m = 0.175; % Kg
disc.A = 0.057; % m^2
disc.d = 2*sqrt(0.057/pi); % 2*sqrt(disc.A/pi); % diameter
disc.Ia = 0.002352; % moment of inertia about the spinning axis
disc.Id = 0.001219; % moment of inertia about the planar axis'

%% helper variables
vel = [xdot ydot zdot];

T_c_Npsi = T_c_N(3,:);

vmag = norm( vel);

r = dot( wD_N_inN, T_c_Npsi);

AdvR = disc.d * r / 2 / vmag; % advance ratio
E_trans = 0.5 * disc.m * vmag*vmag; % translational energy
E_rot = 0.5 * disc.Ia * gammadot*gammadot; % rotational energy

== matlab function hummel_and_hubbard/flatball-6dof/calc-Xdot/calc-THdot ==
  data: X input; M input; THdot output
function THdot   = f_rot( X, M)
% flatball equations of motion - NED (north-east-down) configuration
%

%% internal states
phi = X(4); theta = X(5); gamma = X(6);
p = X(10); q = X(11); r = X(12);

THdot = zeros(1,6);

%% define non-aerodynamic parameters
disc = struct;
disc.Ia = 0.002352; % moment of inertia about the spinning axis
disc.Id = 0.001219; % moment of inertia about the planar axis'

%% helper variables
sin_theta = sin( theta);
cos_theta = cos( theta);

%% add in external forces and moments here
phidotdot = (M(1) + disc.Id*q*p*sin_theta - disc.Ia*q*(p*sin_theta+r) + disc.Id*q*p*sin_theta)/disc.Id/cos_theta; 
thetadotdot = (M(2) + disc.Ia*p*cos_theta*(p*sin_theta +r) - disc.Id*p*p*cos_theta*sin_theta)/disc.Id;
gammadotdot = (M(3) - disc.Ia*(r*sin_theta + q*p*cos_theta))/disc.Ia;

% bug in hummels report?
% gammadotdot = (M(3) - disc.Ia*(phidotdot*sin_theta + thetadot*phidot*cos_theta))/disc.Ia;
% bug in hummels report?
% w/phidotdot term, there is no decay in gammadot
% w/out gammadot term - there is no decay in gammadot
% NOTE: w/it, the decay is too agressive
% FIXME: investigate why this term is necessary for more appropriate
% spindown (based on my data)

%%
THdot(1) = p;
THdot(2) = q;
THdot(3) = r;

THdot(4) = phidotdot;
THdot(5) = thetadotdot;
THdot(6) = gammadotdot;

== matlab function hummel_and_hubbard/flatball-6dof/calc-F-M/calc-alpha/calc-alpha ==
  data: X input; alpha output; T_c_N input
function alpha  = f( X, T_c_N)
%% internal states
u = X(7); v = X(8); w = X(9);

%% helper variables
T_c_Npsi = T_c_N(3,:);

vel = [u v w];
vc3 = dot( vel, T_c_Npsi);
v_N = [ vel - vc3*T_c_Npsi];

alpha = atan( vc3 / norm( v_N)); % angle of attack

== matlab function hummel_and_hubbard/flatball-6dof/calc-F-M/calc-F/X-to-vel ==
  data: X input; vel output
function vel = fcn( X)
u = X(7); v = X(8); w = X(9);
vel = [u v w];

== matlab function hummel_and_hubbard/flatball-6dof/calc-F-M/calc-F/calc-F ==
  data: vel input; F output; T_c_N input; Fg_N input; CLift input; CDrag input; q_inf_times_S input; lift output; drag output; vmag output
function [F, lift, drag, vmag] = fcn( vel, T_c_N, Fg_N, CLift, CDrag, q_inf_times_S)
%%
T_c_Npsi = T_c_N(3,:);

vc3 = dot( vel, T_c_Npsi);
v_N = [ vel - vc3*T_c_Npsi];
vmag = norm( vel);
uvel = vel / vmag;
uv_N = v_N / norm( v_N);
u_lat = cross( T_c_Npsi, uv_N);

lift = CLift * q_inf_times_S;
ulift = -cross( uvel, u_lat);

drag = CDrag * q_inf_times_S;
udrag = -uvel;

Faero = lift*ulift + drag*udrag;

F = Faero' + Fg_N;

== matlab function hummel_and_hubbard/flatball-6dof/calc-F-M/calc-F/q-inf/X-to-vel ==
  data: X input; vel output
function vel = fcn( X)
u = X(7); v = X(8); w = X(9);
vel = [u v w];

== matlab function hummel_and_hubbard/flatball-6dof/calc-F-M/calc-F/q-inf/vector-norm ==
  data: vec input; norm output
function norm = fcn( vec)

norm = sqrt( vec(1)*vec(1) + vec(2)*vec(2) + vec(3)*vec(3));

== matlab function hummel_and_hubbard/flatball-6dof/calc-F-M/calc-M/X-to-vel ==
  data: X input; vel output
function vel = fcn( X)
u = X(7); v = X(7); w = X(9);
vel = [u v w];

== matlab function hummel_and_hubbard/flatball-6dof/calc-F-M/calc-M/calc-M ==
  data: vel input; M output; T_c_N input; wD_N_inN input; q_inf_times_Sd input; CMpitch input; p output; q output; r output
function [M, p, q, r] = fcn( vel, T_c_N, wD_N_inN, q_inf_times_Sd, CMpitch)
%% define ambient parameters
amb.g = 9.81; % m/s^2
amb.rho = 1.23; % Kg/m^3

%% define non-aerodynamic parameters
disc = struct;
disc.m = 0.175; % Kg
disc.A = 0.057; % m^2
disc.d = 2*sqrt(0.057/pi); % 2*sqrt(disc.A/pi); % diameter
disc.Ia = 0.002352; % moment of inertia about the spinning axis
disc.Id = 0.001219; % moment of inertia about the planar axis'

%% best fit coefficients - copied to/from init script!
disc.CNr = -3e-5;
disc.CMq= -1e-3;
disc.CRr = 5e-4;
disc.CRp = -1e-2;

%% helper variables
T_c_Npsi = T_c_N(3,:);

vc3 = dot( vel, T_c_Npsi);
v_N = [ vel - vc3*T_c_Npsi];

uv_N = v_N / norm( v_N);
u_lat = cross( T_c_Npsi, uv_N);

p = dot( wD_N_inN, uv_N);
q = dot( wD_N_inN, u_lat);
r = dot( wD_N_inN, T_c_Npsi);

%% aerodynamic forces and moments in N reference frame
% - is this original and if so, wtf is the sqrt() business about?
% Mv_N = q_inf_times_Sd * (sqrt(disc.d/amb.g)*disc.CRr*r + disc.CRp*p) * uv_N;
% Mpitch = q_inf_times_Sd * (CMpitch + disc.CMq * q) * u_lat;
% Mspin = [0 0 1] .* disc.CNr*r * q_inf_times_Sd;
% M = T_c_N*Mv_N' + T_c_N*Mpitch' + Mspin';

%% aerodynamic forces and moments in N reference frame
M_roll = q_inf_times_Sd * (disc.CRr*r + disc.CRp*p) * uv_N;
M_pitch = q_inf_times_Sd * (CMpitch + disc.CMq*q) * u_lat;
M_yaw = [0 0 1] .* (q_inf_times_Sd * disc.CNr * r);
M = T_c_N*M_roll' + T_c_N*M_pitch' + M_yaw';

== matlab function hummel_and_hubbard/flatball-6dof/calc-F-M/calc-M/q-inf/X-to-vel ==
  data: X input; vel output
function vel = fcn( X)
u = X(7); v = X(7); w = X(9);
vel = [u v w];

== matlab function hummel_and_hubbard/flatball-6dof/calc-F-M/calc-M/q-inf/vector-norm ==
  data: vec input; norm output
function norm = fcn( vec)

norm = sqrt( vec(1)*vec(1) + vec(2)*vec(2) + vec(3)*vec(3));

== matlab function hummel_and_hubbard/flatball-6dof/calc-F-M/rotations/X-to-T_c_N ==
  data: X input; T_c_N output
function T_c_N  = f( X)
%% internal states
phi = X(4); theta = X(5);

%% helper variables
sin_theta = sin( theta);
cos_theta = cos( theta);
sin_phi = sin( phi);
cos_phi = cos(phi);

T_c_N = [
    cos_theta sin_theta*sin_phi -sin_theta*cos_phi;
    0 cos_phi sin_phi;
    sin_theta -cos_theta*sin_phi cos_theta*cos_phi
    ];

== matlab function hummel_and_hubbard/flatball-6dof/calc-F-M/lab/helpers/Subsystem1/transformation-matrices/Ta ==
  data: TH input; M output
function M  = Ta( TH)
% transformation matrix
%
phi = TH(1); theta = TH(2); psi = TH(3);

cos_theta = cos( theta);
cos_phi = cos( phi);
cos_psi = cos( psi);
sin_phi = sin( phi);
sin_theta = sin( theta);
sin_psi = sin( psi);

M = [ ...
    cos_theta*cos_psi sin_phi*sin_theta*cos_phi-cos_phi*sin_psi cos_phi*sin_theta*cos_psi+sin_phi*sin_psi;
    cos_theta*sin_psi sin_phi*sin_theta*sin_psi+cos_phi*cos_psi cos_phi*sin_theta*sin_psi-sin_phi*cos_psi;
    -sin_theta sin_phi*cos_theta cos_phi*cos_theta
    ];

% tan_theta = tan( theta);
% sec_theta = sec( theta);
% transform_r_phi_thea_psi = [
%     1 sin_phi*tan_theta cos_phi*tan_theta
%     0 cos_phi -sin_phi
%     0 sin_phi*sec_theta cos_phi*sec_theta
%     ];

== matlab function hummel_and_hubbard/flatball-6dof/calc-F-M/rotations/X-to-wD_N_inC ==
  data: X input; wD_N_inC output
function wD_N_inC  = f( X)
%% internal states
theta = X(5);
p = X(10); q = X(11); r = X(12);

%% helper variables
sin_theta = sin( theta);
cos_theta = cos( theta);

wD_N_inC = [p*cos_theta q p*sin_theta+r];

== matlab function hummel_and_hubbard/flatball-6dof/calc-F-M/calc-M/internals ==
  data: X input; AdvR output; E_trans output; E_rot output; T_c_N input; wD_N_inN input
function [ AdvR, E_trans, E_rot]  = internals( X, T_c_N, wD_N_inN)
%% internal states
% x = X(1); y = X(2); z = X(3);
u = X(7); v = X(8); w = X(9);

% phi = X(4); theta = X(5); gamma = X(6);
phidot = X(10); thetadot = X(11); gammadot = X(12);

%% define non-aerodynamic parameters
disc = struct;
disc.m = 0.175; % Kg
disc.A = 0.057; % m^2
disc.d = 2*sqrt(0.057/pi); % 2*sqrt(disc.A/pi); % diameter
disc.Ia = 0.002352; % moment of inertia about the spinning axis
disc.Id = 0.001219; % moment of inertia about the planar axis'

%% helper variables
vel = [u v w];

T_c_Npsi = T_c_N(3,:);

vmag = norm( vel);

r = dot( wD_N_inN, T_c_Npsi);

AdvR = disc.d * abs(r) / 2 / vmag; % advance ratio
E_trans = 0.5 * disc.m * vmag*vmag; % translational energy
E_rot = 0.5 * disc.Ia * gammadot*gammadot; % rotational energy

== matlab function hummel_and_hubbard/flatball-6dof/lab/eml-6dof/aero-coefficients ==
  data: X2dot input; alpha3 output; CX output; CTH output; X3dot input; TH3dot input
function [alpha3, CX, CTH] = flatball_6dof(X2dot, X3dot, TH3dot)
%% define ambient conditions
amb.g = 9.7935; % m/s^2
amb.rho = 1.23; % Kg/m^3
%% define flatball (aka - frisbee)

% non-aerodynamic parameters
disc = struct;
disc.m = 0.175; % Kg
disc.I = [0.001219 0 0; 0 0.001219 0; 0 0 0.002352];
disc.c = 0.275;             % Reference chord length (m)
disc.S = pi*(0.275/2)^2;   % Reference area (m^2)

% define flatball aerodynamic properties
disc.alpha0 = -0.052;
disc.CD0 = 0.085;
disc.CDa = 3.30;
disc.CL0 = 0.13;
disc.CLa = 3.09;
disc.CLp = -1.30;
disc.CM0 = -0.01;
disc.CMa = 0.057;
disc.CMq = -1.40;
disc.CNr = -3e-2;

    % calculate aerodynamic coefficients
    u3 = X3dot(1); w3 = X3dot(3);
    p3 = TH3dot(1); q3 = TH3dot(2); r3 = TH3dot(3);
    v_inf = norm( X2dot);

    alpha3 = atan2( w3, u3);                    % angle of attack
    
    CDrag = Cdrag_fcn( alpha3, disc);
    CSide = Cside_fcn( r3, v_inf);
    CLift = Clift_fcn( alpha3, disc);

    CL = CL_fcn( p3, v_inf, disc);
    CM = CM_fcn( alpha3, q3, v_inf, disc);
    CN = CN_fcn( r3, v_inf, disc);

    CX = [-CDrag CSide -CLift];
    CTH = [CL CM CN];
end

function C = Cdrag_fcn( alpha3, disc)
    C = disc.CD0 + disc.CDa * (alpha3 - disc.alpha0)^2;
end

function C = Clift_fcn( alpha3, disc)
    C = disc.CL0 + disc.CLa * alpha3;
end

function C = Cside_fcn( r3, vinf)
    C = -r3 * vinf * 0;                         % <-- 0 == no side force
end

function C = CL_fcn( p3, vinf, disc)
    C = disc.CLp * p3 * disc.c / (2 * vinf);
end

function C = CM_fcn( alpha, q3, vinf, disc)
    C = disc.CM0 + disc.CMa * alpha;
    C = C + (disc.CMq * q3 * disc.c / (2 * vinf));
end

function C = CN_fcn( r3, vinf, disc)
    C = disc.CNr * r3 * disc.c / (2 * vinf);
end

== matlab function hummel_and_hubbard/flatball-6dof/lab/eml-6dof/body-accelerations ==
  data: X2dotdot output; TH2dotdot output; X2dot input; TH2dot input; F2 input; M2 input
function [X2dotdot, TH2dotdot] = flatball_6dof( X2dot, TH2dot, F2, M2)
%% define flatball (aka - frisbee)

% non-aerodynamic parameters
disc = struct;
disc.m = 0.175; % Kg
disc.I = [0.001219 0 0; 0 0.001219 0; 0 0 0.002352];
disc.c = 0.275;             % Reference chord length (m)
disc.S = pi*(0.275/2)^2;   % Reference area (m^2)

    % calculate body accelerations
    p = TH2dot(1); q = TH2dot( 2); r = TH2dot(3);
    w_tilde = [0 -r q; r 0 -p; -q p 0];
    X2dotdot = (F2 ./ disc.m ) - (w_tilde * X2dot);
    TH2dotdot = disc.I^-1 * (M2 - w_tilde * disc.I * TH2dot);
end

== matlab function hummel_and_hubbard/flatball-6dof/lab/eml-6dof/body-force-and-moments ==
  data: F2 output; M2 output; alpha3 input; beta2 input; Ta12 input; F4 input; M4 input
function [F2, M2] = flatball_6dof( alpha3, beta2, Ta12, F4, M4)
%% define ambient conditions
amb.g = 9.7935; % m/s^2
%% define flatball (aka - frisbee)

% non-aerodynamic parameters
disc = struct;
disc.m = 0.175; % Kg

    % calculate forces and moments
    Ta32 = Ta( [0 0 beta2]);
    Ta34 = Ta( [0 alpha3 0]);
    Ta43 = Ta34';
    
    F2aero = Ta43 * Ta32 * F4;
    mg = (disc.m .* [0 0 amb.g]');
    F2 = F2aero + Ta12 * mg;                    % F2
    M2 = Ta43 * Ta32 * M4;                      % M2
end

function T = Ta( TH) %(phi, theta, psi)
    phi = TH(1); theta = TH(2); psi = TH(3);
    T = [
        cos(theta)*cos(psi), sin(phi)*sin(theta)*cos(psi) - cos(phi)*sin(psi), cos(phi)*sin(theta)*cos(psi) + sin(phi)*sin(psi);
        cos(theta)*sin(psi), sin(phi)*sin(theta)*sin(psi) + cos(phi)*cos(psi), cos(phi)*sin(theta)*sin(psi) - sin(phi)*cos(psi);
        -sin(theta), -sin(phi)*cos(theta), cos(phi)*cos(theta)
        ];
end

== matlab function hummel_and_hubbard/flatball-6dof/lab/eml-6dof/earth-reference ==
  data: X1dot output; TH1dot output; Ta21 output; TH1 input; X2dot input; TH2dot input
function [X1dot, TH1dot, Ta21] = flatball_6dof(TH1, X2dot, TH2dot)
    %phi = TH1(1); theta = TH1(2); psi = TH1(3);
    %TH = [phi theta psi];
    Ta21 = Ta( TH1);
    Tr21 = Tr( TH1);

    X1dot = Ta21 * X2dot;                       % X1-dot
    TH1dot = Tr21 * TH2dot;                     % TH1-dotend
end

function T = Ta( TH) %(phi, theta, psi)
    phi = TH(1); theta = TH(2); psi = TH(3);
    T = [
        cos(theta)*cos(psi), sin(phi)*sin(theta)*cos(psi) - cos(phi)*sin(psi), cos(phi)*sin(theta)*cos(psi) + sin(phi)*sin(psi);
        cos(theta)*sin(psi), sin(phi)*sin(theta)*sin(psi) + cos(phi)*cos(psi), cos(phi)*sin(theta)*sin(psi) - sin(phi)*cos(psi);
        -sin(theta), -sin(phi)*cos(theta), cos(phi)*cos(theta)
        ];
end

function T = Tr( TH) %(phi, theta, psi)
    phi = TH(1); theta = TH(2); % psi = TH(3);
    T = [
        1, sin(phi)*tan(theta), cos(phi)*tan(theta);
        0, cos(phi), -sin(phi);
        0, sin(phi)*sec(theta), cos(phi)*sec(theta)
        ];
end

== matlab function hummel_and_hubbard/flatball-6dof/lab/eml-6dof/side-slip-reference ==
  data: X3dot output; TH3dot output; beta2 output; X2dot input; TH2dot input
function [X3dot, TH3dot, beta2] = flatball_6dof(X2dot, TH2dot)
    % calculate zero sideslip variables
    u2 = X2dot(1); v2 = X2dot(2);
    beta2 = atan2( v2, u2);                     % sideslip angle
    
    Ta32 = Ta( [0 0 beta2]);
    Ta23 = Ta32';

    X3dot = Ta23 * X2dot;                       % X3-dot
    TH3dot = Ta23 * TH2dot;                     % TH3-dot
end

function T = Ta( TH) %(phi, theta, psi)
    phi = TH(1); theta = TH(2); psi = TH(3);
    T = [
        cos(theta)*cos(psi), sin(phi)*sin(theta)*cos(psi) - cos(phi)*sin(psi), cos(phi)*sin(theta)*cos(psi) + sin(phi)*sin(psi);
        cos(theta)*sin(psi), sin(phi)*sin(theta)*sin(psi) + cos(phi)*cos(psi), cos(phi)*sin(theta)*sin(psi) - sin(phi)*cos(psi);
        -sin(theta), -sin(phi)*cos(theta), cos(phi)*cos(theta)
        ];
end
